simulink model "lab11"  (R2021b)
settings: Solver=VariableStepAuto  StartTime=0.0  StopTime=10.0  RelTol=1e-3
values from neighbouring files (symbols this model uses):
  x0 = X2(:,m)    [phase_surface.m]    (also in phase_surface2.m)
undefined symbols (not defined in the file or in its folder): b, c, d
settings Model: Creator=roman  LastModifiedBy=roman

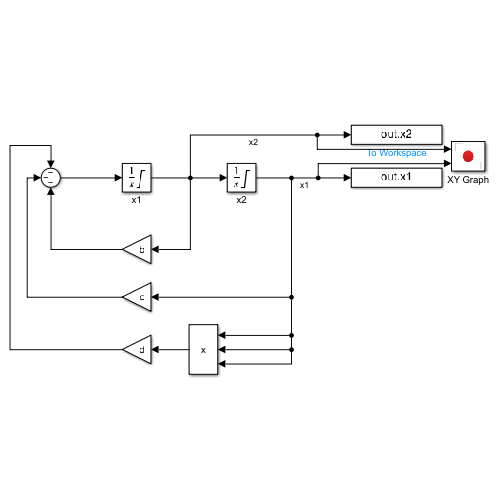
[thumbnail: Simulink's stored preview of the top-level diagram]
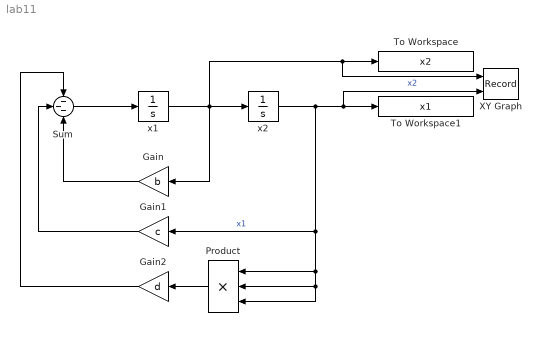
== system lab11 ==
  Gain : Gain  Gain=b
  Gain1 : Gain  Gain=c
  Gain2 : Gain  Gain=d
  Product : Product  Inputs=3
  Sum : Sum  Inputs=---
  To Workspace : ToWorkspace  VariableName=x2  SampleTime=-1
  To Workspace1 : ToWorkspace  VariableName=x1  SampleTime=-1
  XY Graph : Record  FileSettingsInternal="{\"entries\":[{\"content\":{\"excelSettings\":{\"content\":{},\"type\":\"Streamout.ExcelSettings\"}},\"type\":\"Streamout.FileSettingStorage\",\"uuid\":\"bb31664e-d593-449c-bbbe-2638a619c356\"}],\"packageUris\":[\"http://schema.mathworks.com/mf0/streamout_blocks/R2020a\"],\"version\":\"1.0\"}"  Layout=[1 1]  SignalsInternal="{\"entries\":[{\"content\":{\"signals\":[{\"content\":{\"blockPath\":[\"lab11/XY Graph\"],\"channel\":[],\"dimensions\":[1],\"domain\":\"lab11/XY Graph\",\"lineColor\":\"#a2142f\",\"plots\":[1],\"port\":1,\"sid\":[\"\"],\"signalID\":21655,\"signalName\":\"x2\"},\"type\":\"RecordBlkView.Signal\",\"uuid\":\"2533a0b5-f5ea-4653-971a-476dd001762d\"},{\"content\":{\"blockPath\":[\"lab11/XY Graph\"],\"channel\":[],\"dimensions\":[1],\"domain\":\"lab11/XY Graph\",\"lineColor\":\"#139fff\",\"plots\":[1],\"port\":2,\"sid\":[\"\"],\"signalID\":21659,\"signalName\":\"x1\"},\"type\":\"RecordBlkView.Signal\",\"uuid\":\"95f6660e-becd-48a6-80af-3cee44cefd58\"}]},\"type\":\"RecordBlkView.InputSignals\",\"uuid\":\"6ff2cd77-10a3-4d57-8a20-28fc6a764225\"}],\"packageUris\":[\"http://schema.mathworks.com/mf0/streamout_blocks/R2020a\"],\"version\":\"1.0\"}"  VisualizationBindings="{\"xyplotplugin\":{\"info\":[{\"series\":[{\"bindingParametersList\":[{\"parameter\":\"X-Axis\",\"signalID\":21655,\"signalName\":\"x2\"},{\"parameter\":\"Y-Axis\",\"signalID\":21659,\"signalName\":\"x1\"}],\"seriesID\":51632}],\"subplotID\":1}]}}"  CompatibilityTag=XY
  x1 : Integrator  InitialCondition=x0(2)  LimitOutput=on  UpperSaturationLimit=2  LowerSaturationLimit=-2
  x2 : Integrator  InitialCondition=x0(1)  LimitOutput=on  UpperSaturationLimit=2  LowerSaturationLimit=-2
  wires:
  Sum/1 -> x1/1
  x1/1 -> XY Graph/1, To Workspace/1, Gain/1, x2/1  "x2"
  Gain/1 -> Sum/3
  Gain1/1 -> Sum/2
  Product/1 -> Gain2/1
  x2/1 -> To Workspace1/1, XY Graph/2, Product/3, Product/2, Product/1, Gain1/1  "x1"
  Gain2/1 -> Sum/1
